simulink model "explicit_rl_fitted"  (R2021a)
settings: Solver=FixedStepAuto  StartTime=0.0  StopTime=inf  FixedStep=0.5  RelTol=1e-3
libraries: robotlib x10
settings Model: Creator=ivory  LastModifiedBy=sprinkle
settings SolverCC: AlgebraicLoopSolver=TrustRegion
settings OptimizationCC: EnhancedBackFolding=on  PassReuseOutputArgsAs=Individual arguments  ZeroExternalMemoryAtStartup=off  ZeroInternalMemoryAtStartup=off  MaxStackSize=64  OptimizeBlockOrder=speed  DifferentSizesBufferReuse=on  OptimizationCustomize=off  EfficientTunableParamExpr=on
settings DebuggingCC: ParameterTunabilityLossMsg=error  SFMachineParentedDataDiag=warning
settings HardwareCC: ProdBitPerPointer=32  ProdBitPerSizeT=32  ProdBitPerPtrDiffT=32  ProdLargestAtomicFloat=None  ProdIntDivRoundTo=Undefined  ProdEndianess=Unspecified  ProdWordSize=32  ProdHWDeviceType=Generic->Unspecified (assume 32-bit Generic)
settings SFSimCC: MATLABDynamicMemAlloc=off  SimTargetLang=C++
settings RTWCC: SystemTargetFile=ert.tlc  HardwareBoard=Robot Operating System (ROS)  TLCOptions="-aInlineSetEventsForThisBaseRateFcn=TLC_FALSE -aSuppressMultiTaskScheduler=TLC_FALSE  -aRateBasedStepFcn=0"  TemplateMakefile=ert_default_tmf  GenerateReport=on  Toolchain=Catkin  IncludeHyperlinkInReport=on  LaunchReport=on  TargetLang=C++  GenerateTraceInfo=on  GenerateTraceReport=on  GenerateTraceReportSl=on  GenerateTraceReportSf=on  GenerateTraceReportEml=on
settings CodeAppCC: ForceParamTrailComments=on  IgnoreCustomStorageClasses=off  OperatorAnnotations=on  SimulinkDataObjDesc=on  SFDataObjDesc=on  InsertBlockDesc=on
settings ERTTargetCC: SupportContinuousTime=on  SupportVariableSizeSignals=on

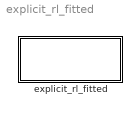
== system explicit_rl_fitted ==
  explicit_rl_fitted : Subsystem

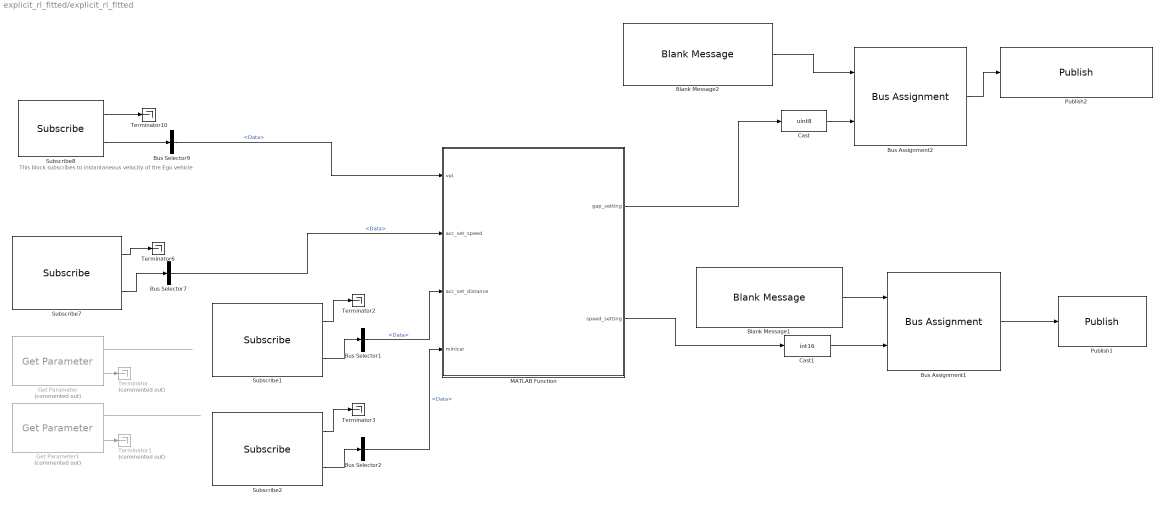
== system explicit_rl_fitted/explicit_rl_fitted ==
  note: This block subscribes to
      | instantaneous velocity of the Ego vehicle
  Blank Message1 : robotlib/Blank Message  messageClass=Message  entityType=std_msgs/Int16  messageType=std_msgs/Int16  SampleTime=inf  legacyBusStruct=off
  Blank Message2 : robotlib/Blank Message  messageClass=Message  entityType=std_msgs/UInt8  messageType=std_msgs/UInt8  SampleTime=inf  legacyBusStruct=off
  Bus Assignment1 : BusAssignment  AssignedSignals=Data
  Bus Assignment2 : BusAssignment  AssignedSignals=Data
  Bus Selector{1..2,7,9} (4 alike) : BusSelector  OutputSignals=Data
  Cast : DataTypeConversion  OutDataTypeStr=uint8
  Cast1 : DataTypeConversion  OutDataTypeStr=int16
  Get Parameter : robotlib/Get Parameter  Commented=on  ParameterSource=Specify your own  ParameterName=target_speed  ParameterType=double  ParameterMaxArrayLength=16  ParameterInitialValue=25.0  SampleTime=-1  ShowErrorCodeOutput=on  ModelName=acc_settings  BlockId=ParamGet_acc_settings_655
      settings: SourceProductBaseCode=RR
  Get Parameter1 : robotlib/Get Parameter  Commented=on  ParameterSource=Specify your own  ParameterName=max_headway  ParameterType=double  ParameterMaxArrayLength=16  ParameterInitialValue=50.0  SampleTime=-1  ShowErrorCodeOutput=on  ModelName=acc_settings  BlockId=ParamGet_acc_settings_657
      settings: SourceProductBaseCode=RR
  MATLAB Function : MATLAB Function  TreatAsAtomicUnit=on
  Publish1 : robotlib/Publish  topicSource=Specify your own  topic=speed_setting  messageType=std_msgs/Int16  legacyBusStruct=off  messageQueueLength=1
  Publish2 : robotlib/Publish  topicSource=Specify your own  topic=target_gap_setting  messageType=std_msgs/UInt8  legacyBusStruct=off  messageQueueLength=1
  Subscribe1 : robotlib/Subscribe  topicSource=Specify your own  topic=acc/set_distance  messageType=std_msgs/Int16  SampleTime=-1  legacyBusStruct=off  messageQueueLength=1
  Subscribe2 : robotlib/Subscribe  topicSource=Specify your own  topic=acc/mini_car  messageType=std_msgs/Int16  SampleTime=-1  legacyBusStruct=off  messageQueueLength=1
  Subscribe7 : robotlib/Subscribe  topicSource=Specify your own  topic=acc/set_speed  messageType=std_msgs/Int16  SampleTime=-1  legacyBusStruct=off  messageQueueLength=1
  Subscribe8 : robotlib/Subscribe  topicSource=Specify your own  topic=vel  messageType=std_msgs/Float64  SampleTime=-1  legacyBusStruct=off  messageQueueLength=1
  Terminator : Terminator  Commented=on
  Terminator1 : Terminator  Commented=on
  Terminator{2..3,6,10} (4 alike) : Terminator
  wires:
  Subscribe8/2 -> Bus Selector9/1
  Subscribe8/1 -> Terminator10/1
  Bus Selector9/1 -> MATLAB Function/1(vel)  "<Data>"
  Subscribe7/1 -> Terminator6/1
  Subscribe7/2 -> Bus Selector7/1
  Get Parameter/1 -> ?
  Get Parameter/2 -> Terminator/1
  Get Parameter1/2 -> Terminator1/1
  Get Parameter1/1 -> ?
  Bus Assignment2/1 -> Publish2/1
  Blank Message2/1 -> Bus Assignment2/1
  MATLAB Function/1(gap_setting) -> Cast/1
  MATLAB Function/2(speed_setting) -> Cast1/1
  Blank Message1/1 -> Bus Assignment1/1
  Bus Assignment1/1 -> Publish1/1
  Cast/1 -> Bus Assignment2/2
  Cast1/1 -> Bus Assignment1/2
  Bus Selector7/1 -> MATLAB Function/2(acc_set_speed)  "<Data>"
  Subscribe1/1 -> Terminator2/1
  Subscribe1/2 -> Bus Selector1/1
  Bus Selector1/1 -> MATLAB Function/3(acc_set_distance)  "<Data>"
  Subscribe2/1 -> Terminator3/1
  Bus Selector2/1 -> MATLAB Function/4(minicar)  "<Data>"
  Subscribe2/2 -> Bus Selector2/1

== matlab function explicit_rl_fitted/MATLAB Function ==
  settings: updateMethod=DISCRETE
  data: vel input; acc_set_speed input; gap_setting output; acc_set_distance input; minicar input; speed_setting output
function [gap_setting, speed_setting] =  get_acc_accel(vel, acc_set_speed, acc_set_distance, minicar)
        %%"""See parent class."""
        KPH_TO_MPH = 0.621371;
        MPH_TO_MS = 0.44704;
        MS_TO_MPH = 1/MPH_TO_MS;
        speed_setting = int16(acc_set_speed * KPH_TO_MPH);
        gap_setting = uint8(acc_set_distance);
        %% base logic:
        % if we are slowing down because we just met a car
        % then we should reduce our 'bars' until we get to one
        % if we are speeding up
        % then we set our bars up to 3 again
        %% first, we make sure our setpoint is 70
        % TODO: make 70 a parameter
        if( acc_set_speed < 70 )
            speed_setting = int16(70);
        else
            %% now set the bars as appropriate
            if (minicar == 0 )
                gap_setting = uint8(3);
            elseif (acc_set_distance > 1 && minicar == 1)
                speed = vel * MS_TO_MPH;
                if ( abs(speed - acc_set_speed) > 5 )
                    gap_setting = uint8(acc_set_distance - 1);
                end
            end
        end
end
